simulink model "ABS"  (R2020b)
settings: Solver=VariableStepAuto  StartTime=0.0  StopTime=10.0  RelTol=1e-3
values from neighbouring files (symbols this model uses):
  ctrl = 1    [parameters.m]
  g = 32.18    [parameters.m]
  m = 50    [parameters.m]
  mu = [0 .4 .8 .97 1.0 .98 .96 .94 .92 .9 .88 .855 .83 .81 .79 .77 .75 .73 .72 .71 .7]    [parameters.m]
  Rr = 15/12    (= 1.25)    [parameters.m]
  slip = (0:.05:1.0)    [parameters.m]
  v0 = 88    [parameters.m]
settings Model: Creator=adity  LastModifiedBy=adity

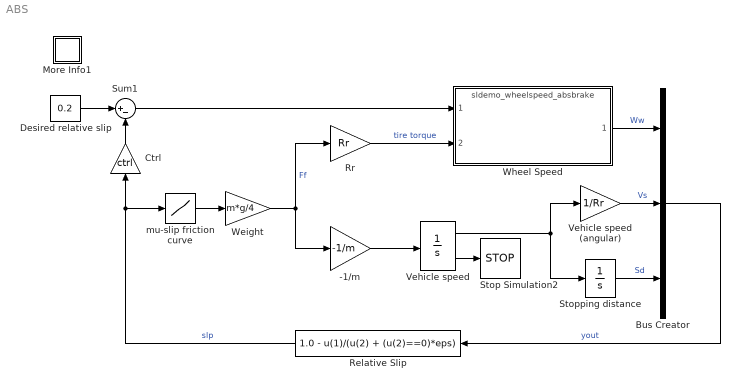
== system ABS ==
  -1/m : Gain  Gain=-1/m  SaturateOnIntegerOverflow=on  OutDataTypeStr=Inherit: Same as input  ParamDataTypeStr=Inherit: Same as input
  Bus Creator : BusCreator  Inputs=3
  Ctrl : Gain  Gain=ctrl  SaturateOnIntegerOverflow=on  OutDataTypeStr=Inherit: Same as input  ParamDataTypeStr=Inherit: Same as input
  Desired relative slip : Constant  Value=0.2
  More Info1 : Subsystem
      settings: OpenFcn=showExample('simulink_automotive/ModelingAnAntiLockBrakingSystemExample')
      mask Display: disp('?')
  Relative Slip : Fcn  Expr=1.0 - u(1)/(u(2) + (u(2)==0)*eps)
  Rr : Gain  Gain=Rr  SaturateOnIntegerOverflow=on  OutDataTypeStr=Inherit: Same as input  ParamDataTypeStr=Inherit: Same as input
  Stop Simulation2 : Stop
  Stopping distance : Integrator  UpperSaturationLimit=1000  LowerSaturationLimit=0
  Sum1 : Sum  Inputs=|+-  InputSameDT=on  SaturateOnIntegerOverflow=on  OutDataTypeStr=Inherit: Same as first input
  Vehicle speed : Integrator  InitialCondition=v0  LimitOutput=on  UpperSaturationLimit=1000  LowerSaturationLimit=0  ShowSaturationPort=on
  Vehicle speed (angular) : Gain  Gain=1/Rr  SaturateOnIntegerOverflow=on  OutDataTypeStr=Inherit: Same as input  ParamDataTypeStr=Inherit: Same as input
  Weight : Gain  Gain=m*g/4  SaturateOnIntegerOverflow=on  OutDataTypeStr=Inherit: Same as input  ParamDataTypeStr=Inherit: Same as input
  Wheel Speed : ModelReference  ModelNameDialog=sldemo_wheelspeed_absbrake  SimulationMode=Normal  ModelReferenceVersion=1.67
  mu-slip friction curve : Lookup_n-D  NumberOfTableDimensions=1  BreakpointsForDimension1=slip  Table=mu  SaturateOnIntegerOverflow=on  InputSameDT=on
  wires:
  mu-slip friction curve/1 -> Weight/1
  Desired relative slip/1 -> Sum1/1
  Sum1/1 -> Wheel Speed/1
  Stopping distance/1 -> Bus Creator/3  "Sd"
  Rr/1 -> Wheel Speed/2  "tire torque"
  Wheel Speed/1 -> Bus Creator/1  "Ww"
  Vehicle speed/1 -> Stopping distance/1, Vehicle speed (angular)/1
  Ctrl/1 -> Sum1/2
  Weight/1 -> -1/m/1, Rr/1  "Ff"
  Relative Slip/1 -> mu-slip friction curve/1, Ctrl/1  "slp"
  Vehicle speed/2 -> Stop Simulation2/1
  Vehicle speed (angular)/1 -> Bus Creator/2  "Vs"
  Bus Creator/1 -> Relative Slip/1  "yout"
  -1/m/1 -> Vehicle speed/1

== system ABS/More Info1 ==
